simulink model "Lab2_model"  (R2023b)
settings: Solver=FixedStepAuto  StartTime=0.0  StopTime=30  FixedStep=.01  RelTol=1e-3
undefined symbols (not defined in the file or in its folder): A, B, C
settings Model: Creator=Connor Emmons  LastModifiedBy=Connor Emmons

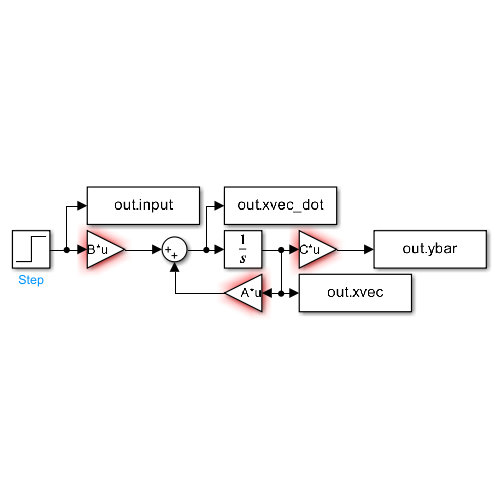
[thumbnail: Simulink's stored preview of the top-level diagram]
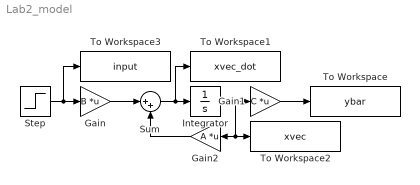
== system Lab2_model ==
  Gain : Gain  Gain=B  Multiplication=Matrix(K*u)
  Gain1 : Gain  Gain=C  Multiplication=Matrix(K*u)
  Gain2 : Gain  Gain=A  Multiplication=Matrix(K*u)
  Integrator : Integrator
  Step : Step  SampleTime=0
  Sum : Sum  Inputs=|++
  To Workspace : ToWorkspace  VariableName=ybar  SampleTime=-1
  To Workspace1 : ToWorkspace  VariableName=xvec_dot  SampleTime=-1
  To Workspace2 : ToWorkspace  VariableName=xvec  SampleTime=-1
  To Workspace3 : ToWorkspace  VariableName=input  SampleTime=-1
  wires:
  Gain/1 -> Sum/1
  Sum/1 -> To Workspace1/1, Integrator/1
  Integrator/1 -> To Workspace2/1, Gain2/1, Gain1/1
  Gain2/1 -> Sum/2
  Gain1/1 -> To Workspace/1
  Step/1 -> To Workspace3/1, Gain/1
